simulink model "valve_test_2"  (R2021a)
settings: Solver=VariableStepAuto  StartTime=0.0  StopTime=100  RelTol=1e-3
undefined symbols (not defined in the file or in its folder): C_1, C_2, C_A_in, C_A_out, C_adj_in, flow_C, flow_C_ratio, flow_noise_var, gamma, p0, p1, p2, p3, p4, P_0, P_cr, P_s, spool_dynamic, spool_valve_time_delay, T, Ts, valve1
settings Model: Creator=artof  LastModifiedBy=artof

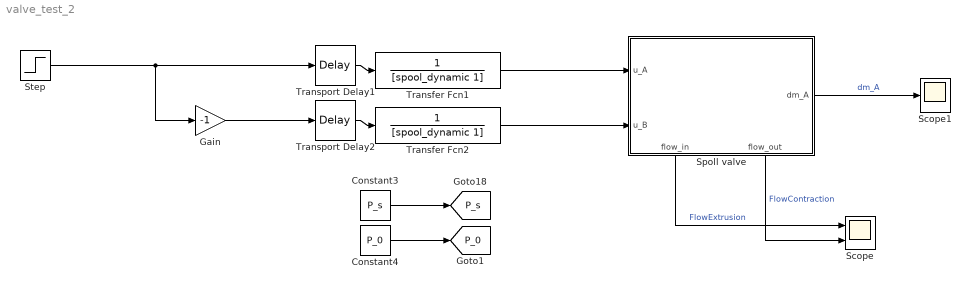
== system valve_test_2 ==
  Constant3 : Constant  Value=P_s
  Constant4 : Constant  Value=P_0
  Gain : Gain  Gain=-1
  Scope : Scope  NumInputPorts=2
  Scope1 : Scope
  Spoll valve : Subsystem
      settings: PortSchema="{\"entries\":[{\"content\":{\"sides\":[{\"content\":{\"connectorIds\":[\"In1\",\"In2\"]},\"type\":\"ConnectorPlacement.EquallySpacedRectSide\",\"uuid\":\"f49fadee-fa9e-4c00-be17-3013d1757a7f\"},{\"content\":{\"connectorIds\":[\"Out1\"],\"side\":\"RIGHT\"},\"type\":\"ConnectorPlacement.EquallySpacedRectSide\",\"uuid\":\"640b0073-0df7-45c7-9e72-cb244187d5a1\"},{\"content\":{\"connectorIds\":[],\"side\":\"TOP\"},\"type\":\"ConnectorPlacement.EquallySpacedRectSide\",\"uuid\":\"42e207d6-f026-4ddf-97dc-8c7968fc41f1\"},{\"content\":{\"connectorIds\":[\"Out2\",\"Out3\"],\"side\":\"BOTTOM\"},\"type\":\"ConnectorPlacement.EquallySpacedRectSide\",\"uuid\":\"eeba3cdd-6d70-46a7-a1e2-c2998fe430fd\"}]},\"type\":\"ConnectorPlacement.EquallySpacedConnector\",\"uuid\":\"e8c5a427-dc83-42b8-9540-729b85904a46\"}],\"packageUris\":[\"http://schema.mathworks.com/mf0/Connector/R2020b\"],\"version\":\"1.0\"}"
  Step : Step  SampleTime=0
  Transfer Fcn1 : TransferFcn  Denominator=[spool_dynamic 1]
  Transfer Fcn2 : TransferFcn  Denominator=[spool_dynamic 1]
  Transport Delay1 : TransportDelay  DelayTime=spool_valve_time_delay
  Transport Delay2 : TransportDelay  DelayTime=spool_valve_time_delay
  tag scope: P_0=global, P_s=global
  wires:
  Transport Delay1/1 -> Transfer Fcn1/1
  Transport Delay2/1 -> Transfer Fcn2/1
  Transfer Fcn2/1 -> Spoll valve/2(u_B)
  Step/1 -> Gain/1, Transport Delay1/1
  Gain/1 -> Transport Delay2/1
  Spoll valve/2(flow_in) -> Scope/1  "FlowExtrusion"
  Spoll valve/3(flow_out) -> Scope/2  "FlowContraction"
  Transfer Fcn1/1 -> Spoll valve/1(u_A)
  Spoll valve/1(dm_A) -> Scope1/1  "dm_A"
  Constant4/1 -> [P_0]
  Constant3/1 -> [P_s]

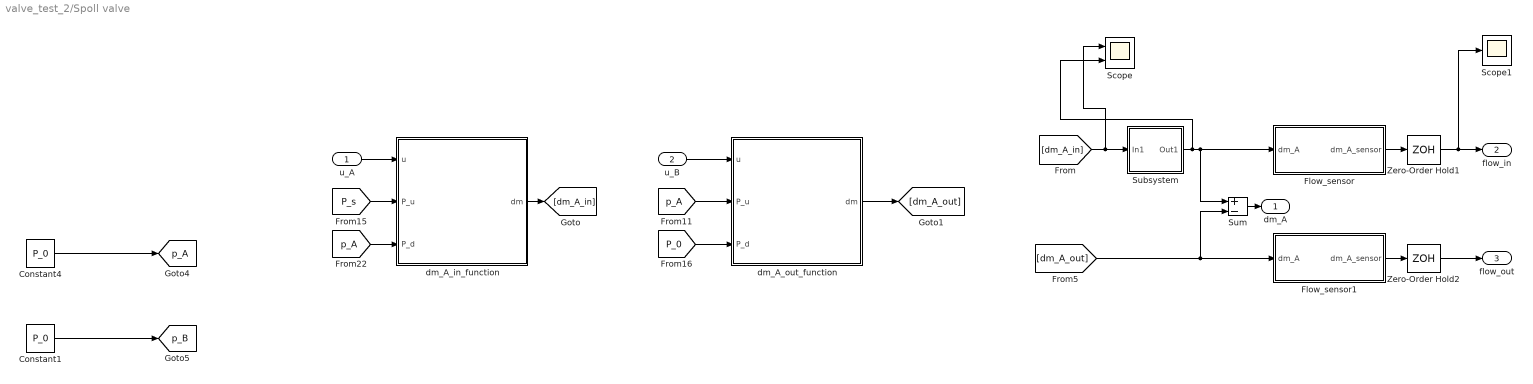
== system valve_test_2/Spoll valve ==
  u_A : Inport
  u_B : Inport  Port=2
  Constant1 : Constant  Value=P_0
  Constant4 : Constant  Value=P_0
  Flow_sensor : MATLAB Function  TreatAsAtomicUnit=on
  Flow_sensor1 : MATLAB Function  TreatAsAtomicUnit=on
  Scope : Scope  NumInputPorts=2
  Scope1 : Scope
  Subsystem : Subsystem
  Sum : Sum  Inputs=+-
  Zero-Order Hold1 : ZeroOrderHold  SampleTime=Ts
  Zero-Order Hold2 : ZeroOrderHold  SampleTime=Ts
  dm_A_in_function : MATLAB Function  TreatAsAtomicUnit=on
  dm_A_out_function : MATLAB Function  TreatAsAtomicUnit=on
  dm_A : Outport
  flow_in : Outport  Port=2
  flow_out : Outport  Port=3
  tag scope: p_A=global, p_B=global
  wires:
  [P_s] -> dm_A_in_function/2(P_u)
  [p_A] -> dm_A_in_function/3(P_d)
  dm_A_in_function/1(dm) -> [dm_A_in]
  dm_A_out_function/1(dm) -> [dm_A_out]
  [p_A] -> dm_A_out_function/2(P_u)
  [P_0] -> dm_A_out_function/3(P_d)
  u_A/1 -> dm_A_in_function/1(u)
  u_B/1 -> dm_A_out_function/1(u)
  [dm_A_in] -> Scope/1, Subsystem/1(In1)
  Sum/1 -> dm_A/1
  Flow_sensor/1(dm_A_sensor) -> Zero-Order Hold1/1
  Flow_sensor1/1(dm_A_sensor) -> Zero-Order Hold2/1
  [dm_A_out] -> Sum/2, Flow_sensor1/1(dm_A)
  Zero-Order Hold1/1 -> Scope1/1, flow_in/1
  Zero-Order Hold2/1 -> flow_out/1
  Subsystem/1(Out1) -> Scope/2, Sum/1, Flow_sensor/1(dm_A)
  Constant4/1 -> [p_A]
  Constant1/1 -> [p_B]

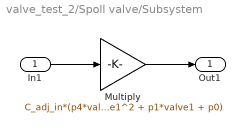
== system valve_test_2/Spoll valve/Subsystem ==
  In1 : Inport
  Multiply : Gain  Gain=C_adj_in*(p4*valve1^4 + p3*valve1^3+p2*valve1^2 + p1*valve1 + p0)
  Out1 : Outport
  wires:
  In1/1 -> Multiply/1
  Multiply/1 -> Out1/1

== matlab function valve_test_2/Spoll valve/Flow_sensor ==
  settings: updateMethod=DISCRETE
  data: dm_A input; dm_A_sensor output; flow_C parameter; flow_C_ratio parameter; flow_noise_var parameter
function dm_A_sensor = fcn(dm_A, flow_C, flow_C_ratio, flow_noise_var)
dm_A_sensor = flow_C*(flow_C_ratio*dm_A + flow_noise_var*rand());

== matlab function valve_test_2/Spoll valve/Flow_sensor1 ==
  settings: updateMethod=DISCRETE
  data: dm_A input; dm_A_sensor output; flow_C parameter; flow_C_ratio parameter; flow_noise_var parameter
function dm_A_sensor = fcn(dm_A, flow_C, flow_C_ratio, flow_noise_var)
dm_A_sensor = flow_C*(flow_C_ratio*dm_A + flow_noise_var*rand());

== matlab function valve_test_2/Spoll valve/dm_A_in_function ==
  data: u input; dm output; P_u input; P_d input; C_A_in parameter; C_1 parameter; C_2 parameter; P_cr parameter; T parameter; gamma parameter
function dm = fcn(u, P_u, P_d, C_A_in, C_1, C_2, P_cr, T, gamma)
if u > 0    
    P_ratio = P_d/P_u;
    if P_ratio <= P_cr && P_ratio >= 0
        dm = u*C_A_in*C_1*P_u/sqrt(T);
    elseif P_ratio > P_cr && P_ratio <= 1
        dm = u*C_A_in*C_2*P_u/sqrt(T)*P_ratio^(1/gamma)*sqrt(1-P_ratio^((gamma-1)/gamma));
    else
        %dm = -u*C_A_in*C_2*P_d/sqrt(T)*(1/P_ratio)^(1/gamma)*sqrt(1-(1/P_ratio)^((gamma-1)/gamma));
        dm = 0;
    end
else
    dm = 0;
end

== matlab function valve_test_2/Spoll valve/dm_A_out_function ==
  data: u input; dm output; P_u input; P_d input; C_A_out parameter; C_1 parameter; P_cr parameter; C_2 parameter; T parameter; gamma parameter
function dm = fcn(u, P_u, P_d, C_A_out, C_1, P_cr, C_2, T, gamma)
if u > 0    
    P_ratio = P_d/P_u;
    if P_ratio <= P_cr && P_ratio >= 0
        dm = u*C_A_out*C_1*P_u/sqrt(T);
    elseif P_ratio > P_cr && P_ratio <= 1
        dm = u*C_A_out*C_2*P_u/sqrt(T)*P_ratio^(1/gamma)*sqrt(1-P_ratio^((gamma-1)/gamma));
    else
        %dm = -u*C_A_out*C_2*P_d/sqrt(T)*(1/P_ratio)^(1/gamma)*sqrt(1-(1/P_ratio)^((gamma-1)/gamma));
        dm = 0;
    end
else
    dm = 0;
end
